simulink model "TEModel"  (Simulink 8.6)
settings: Solver=ode1  SolverMode=SingleTasking  StartTime=0.0  StopTime=72  FixedStep=Ts_base  MaxStep=Ts_base  MinStep=1e-6  RelTol=1e-6
PreLoadFcn:
  | initModel
StopFcn:
  | TEplot
undefined symbols (not defined in the file): Ts_base, Ts_save
libraries: TElib x45
(part 7 of 9)

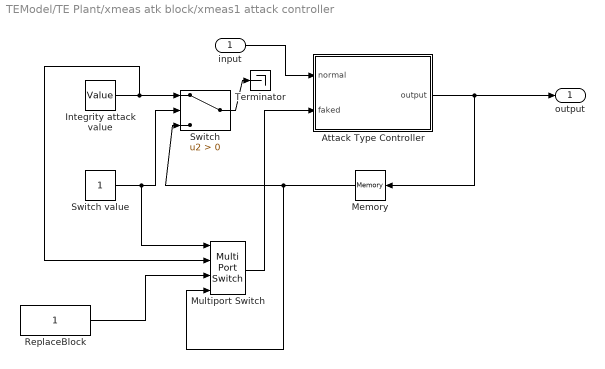
== system TEModel/TE Plant/xmeas atk block/xmeas1 attack controller ==
  input : Inport
  Attack Type Controller : Subsystem  Variant=on  OverrideUsingVariant=normal_forward_controller  mask{atkMode=No attack, start=1, duration=duration}
      mask prompts: atkMode "Attack Mode:"
      mask TypeOptions atkMode: No attack | Step attack | Interval attack | Periodical attack
      mask Callback atkMode:
      | switch get_param(gcb,'atkMode');
      |     case 'Step attack'
      |         set_param(gcb, 'OverrideUsingVariant', 'step_forward_controller');
      |     case 'Interval attack'
      |         set_param(gcb, 'OverrideUsingVariant', 'interval_forward_controller');
      |     case 'Periodical attack'
      |         set_param(gcb, 'OverrideUsingVariant', 'periodical_forward_controller');
      |     otherwise
      |         set_param(gcb, 'OverrideUsingVariant', 'normal_forward_controller');
      | end
      mask Display: eval(get_param([gcb '/' strrep(get_param(gcb, 'ActiveVariant'), '_', ' ')], 'MaskDisplay'));
  Integrity attack value : Constant  Value=Value
  Memory : Memory
  Multiport Switch : MultiPortSwitch
  ReplaceBlock : Constant
  Switch : Switch  Criteria=u2 > Threshold
  Switch value : Constant
  Terminator : Terminator
  output : Outport
  wires:
  Integrity attack value/1 -> Multiport Switch/2, Switch/1
  Attack Type Controller/1(output) -> Memory/1, output/1
  Switch value/1 -> Multiport Switch/1, Switch/2
  input/1 -> Attack Type Controller/1(normal)
  Memory/1 -> Multiport Switch/4, Switch/3
  Multiport Switch/1 -> Attack Type Controller/2(faked)
  Switch/1 -> Terminator/1
  ReplaceBlock/1 -> Multiport Switch/3

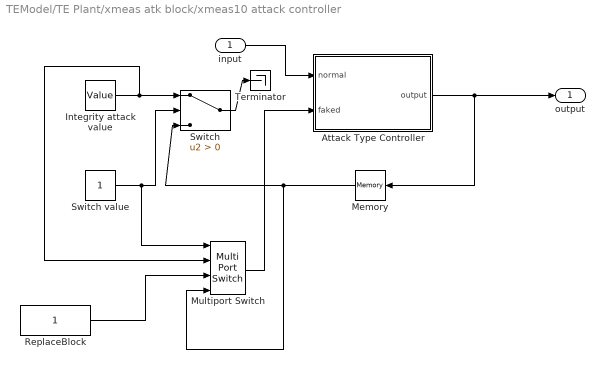
== system TEModel/TE Plant/xmeas atk block/xmeas10 attack controller ==
  input : Inport
  Attack Type Controller : Subsystem  Variant=on  OverrideUsingVariant=normal_forward_controller  mask{atkMode=No attack, start=1, duration=duration}
      mask prompts: atkMode "Attack Mode:"
      mask TypeOptions atkMode: No attack | Step attack | Interval attack | Periodical attack
      mask Callback atkMode:
      | switch get_param(gcb,'atkMode');
      |     case 'Step attack'
      |         set_param(gcb, 'OverrideUsingVariant', 'step_forward_controller');
      |     case 'Interval attack'
      |         set_param(gcb, 'OverrideUsingVariant', 'interval_forward_controller');
      |     case 'Periodical attack'
      |         set_param(gcb, 'OverrideUsingVariant', 'periodical_forward_controller');
      |     otherwise
      |         set_param(gcb, 'OverrideUsingVariant', 'normal_forward_controller');
      | end
      mask Display: eval(get_param([gcb '/' strrep(get_param(gcb, 'ActiveVariant'), '_', ' ')], 'MaskDisplay'));
  Integrity attack value : Constant  Value=Value
  Memory : Memory
  Multiport Switch : MultiPortSwitch
  ReplaceBlock : Constant
  Switch : Switch  Criteria=u2 > Threshold
  Switch value : Constant
  Terminator : Terminator
  output : Outport
  wires:
  Integrity attack value/1 -> Multiport Switch/2, Switch/1
  Attack Type Controller/1(output) -> Memory/1, output/1
  Switch value/1 -> Multiport Switch/1, Switch/2
  input/1 -> Attack Type Controller/1(normal)
  Memory/1 -> Multiport Switch/4, Switch/3
  Multiport Switch/1 -> Attack Type Controller/2(faked)
  Switch/1 -> Terminator/1
  ReplaceBlock/1 -> Multiport Switch/3

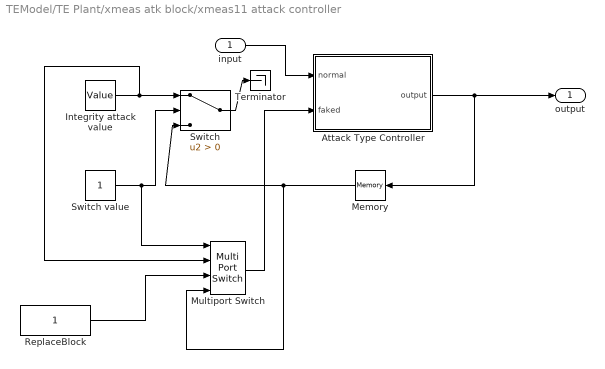
== system TEModel/TE Plant/xmeas atk block/xmeas11 attack controller ==
  input : Inport
  Attack Type Controller : Subsystem  Variant=on  OverrideUsingVariant=normal_forward_controller  mask{atkMode=No attack, start=1, duration=duration}
      mask prompts: atkMode "Attack Mode:"
      mask TypeOptions atkMode: No attack | Step attack | Interval attack | Periodical attack
      mask Callback atkMode:
      | switch get_param(gcb,'atkMode');
      |     case 'Step attack'
      |         set_param(gcb, 'OverrideUsingVariant', 'step_forward_controller');
      |     case 'Interval attack'
      |         set_param(gcb, 'OverrideUsingVariant', 'interval_forward_controller');
      |     case 'Periodical attack'
      |         set_param(gcb, 'OverrideUsingVariant', 'periodical_forward_controller');
      |     otherwise
      |         set_param(gcb, 'OverrideUsingVariant', 'normal_forward_controller');
      | end
      mask Display: eval(get_param([gcb '/' strrep(get_param(gcb, 'ActiveVariant'), '_', ' ')], 'MaskDisplay'));
  Integrity attack value : Constant  Value=Value
  Memory : Memory
  Multiport Switch : MultiPortSwitch
  ReplaceBlock : Constant
  Switch : Switch  Criteria=u2 > Threshold
  Switch value : Constant
  Terminator : Terminator
  output : Outport
  wires:
  Integrity attack value/1 -> Multiport Switch/2, Switch/1
  Attack Type Controller/1(output) -> Memory/1, output/1
  Switch value/1 -> Multiport Switch/1, Switch/2
  input/1 -> Attack Type Controller/1(normal)
  Memory/1 -> Multiport Switch/4, Switch/3
  Multiport Switch/1 -> Attack Type Controller/2(faked)
  Switch/1 -> Terminator/1
  ReplaceBlock/1 -> Multiport Switch/3

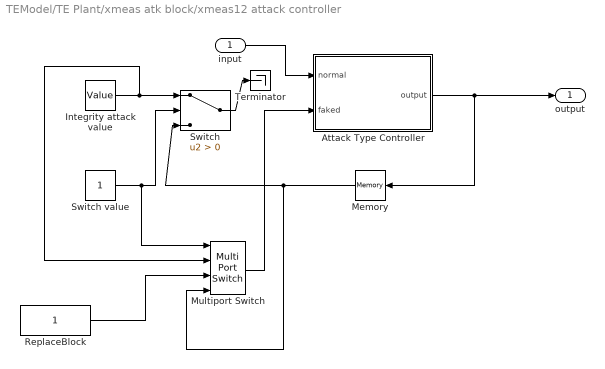
== system TEModel/TE Plant/xmeas atk block/xmeas12 attack controller ==
  input : Inport
  Attack Type Controller : Subsystem  Variant=on  OverrideUsingVariant=normal_forward_controller  mask{atkMode=No attack, start=1, duration=duration}
      mask prompts: atkMode "Attack Mode:"
      mask TypeOptions atkMode: No attack | Step attack | Interval attack | Periodical attack
      mask Callback atkMode:
      | switch get_param(gcb,'atkMode');
      |     case 'Step attack'
      |         set_param(gcb, 'OverrideUsingVariant', 'step_forward_controller');
      |     case 'Interval attack'
      |         set_param(gcb, 'OverrideUsingVariant', 'interval_forward_controller');
      |     case 'Periodical attack'
      |         set_param(gcb, 'OverrideUsingVariant', 'periodical_forward_controller');
      |     otherwise
      |         set_param(gcb, 'OverrideUsingVariant', 'normal_forward_controller');
      | end
      mask Display: eval(get_param([gcb '/' strrep(get_param(gcb, 'ActiveVariant'), '_', ' ')], 'MaskDisplay'));
  Integrity attack value : Constant  Value=Value
  Memory : Memory
  Multiport Switch : MultiPortSwitch
  ReplaceBlock : Constant
  Switch : Switch  Criteria=u2 > Threshold
  Switch value : Constant
  Terminator : Terminator
  output : Outport
  wires:
  Integrity attack value/1 -> Multiport Switch/2, Switch/1
  Attack Type Controller/1(output) -> Memory/1, output/1
  Switch value/1 -> Multiport Switch/1, Switch/2
  input/1 -> Attack Type Controller/1(normal)
  Memory/1 -> Multiport Switch/4, Switch/3
  Multiport Switch/1 -> Attack Type Controller/2(faked)
  Switch/1 -> Terminator/1
  ReplaceBlock/1 -> Multiport Switch/3

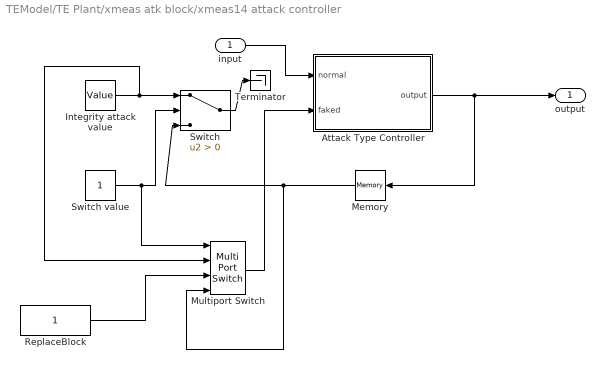
== system TEModel/TE Plant/xmeas atk block/xmeas14 attack controller ==
  input : Inport
  Attack Type Controller : Subsystem  Variant=on  OverrideUsingVariant=normal_forward_controller  mask{atkMode=No attack, start=1, duration=duration}
      mask prompts: atkMode "Attack Mode:"
      mask TypeOptions atkMode: No attack | Step attack | Interval attack | Periodical attack
      mask Callback atkMode:
      | switch get_param(gcb,'atkMode');
      |     case 'Step attack'
      |         set_param(gcb, 'OverrideUsingVariant', 'step_forward_controller');
      |     case 'Interval attack'
      |         set_param(gcb, 'OverrideUsingVariant', 'interval_forward_controller');
      |     case 'Periodical attack'
      |         set_param(gcb, 'OverrideUsingVariant', 'periodical_forward_controller');
      |     otherwise
      |         set_param(gcb, 'OverrideUsingVariant', 'normal_forward_controller');
      | end
      mask Display: eval(get_param([gcb '/' strrep(get_param(gcb, 'ActiveVariant'), '_', ' ')], 'MaskDisplay'));
  Integrity attack value : Constant  Value=Value
  Memory : Memory
  Multiport Switch : MultiPortSwitch
  ReplaceBlock : Constant
  Switch : Switch  Criteria=u2 > Threshold
  Switch value : Constant
  Terminator : Terminator
  output : Outport
  wires:
  Integrity attack value/1 -> Multiport Switch/2, Switch/1
  Attack Type Controller/1(output) -> Memory/1, output/1
  Switch value/1 -> Multiport Switch/1, Switch/2
  input/1 -> Attack Type Controller/1(normal)
  Memory/1 -> Multiport Switch/4, Switch/3
  Multiport Switch/1 -> Attack Type Controller/2(faked)
  Switch/1 -> Terminator/1
  ReplaceBlock/1 -> Multiport Switch/3

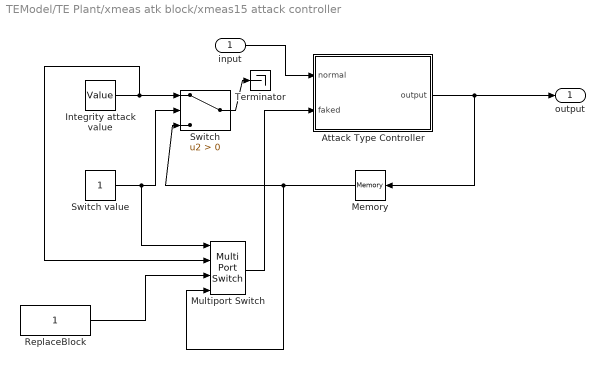
== system TEModel/TE Plant/xmeas atk block/xmeas15 attack controller ==
  input : Inport
  Attack Type Controller : Subsystem  Variant=on  OverrideUsingVariant=normal_forward_controller  mask{atkMode=No attack, start=1, duration=duration}
      mask prompts: atkMode "Attack Mode:"
      mask TypeOptions atkMode: No attack | Step attack | Interval attack | Periodical attack
      mask Callback atkMode:
      | switch get_param(gcb,'atkMode');
      |     case 'Step attack'
      |         set_param(gcb, 'OverrideUsingVariant', 'step_forward_controller');
      |     case 'Interval attack'
      |         set_param(gcb, 'OverrideUsingVariant', 'interval_forward_controller');
      |     case 'Periodical attack'
      |         set_param(gcb, 'OverrideUsingVariant', 'periodical_forward_controller');
      |     otherwise
      |         set_param(gcb, 'OverrideUsingVariant', 'normal_forward_controller');
      | end
      mask Display: eval(get_param([gcb '/' strrep(get_param(gcb, 'ActiveVariant'), '_', ' ')], 'MaskDisplay'));
  Integrity attack value : Constant  Value=Value
  Memory : Memory
  Multiport Switch : MultiPortSwitch
  ReplaceBlock : Constant
  Switch : Switch  Criteria=u2 > Threshold
  Switch value : Constant
  Terminator : Terminator
  output : Outport
  wires:
  Integrity attack value/1 -> Multiport Switch/2, Switch/1
  Attack Type Controller/1(output) -> Memory/1, output/1
  Switch value/1 -> Multiport Switch/1, Switch/2
  input/1 -> Attack Type Controller/1(normal)
  Memory/1 -> Multiport Switch/4, Switch/3
  Multiport Switch/1 -> Attack Type Controller/2(faked)
  Switch/1 -> Terminator/1
  ReplaceBlock/1 -> Multiport Switch/3

== system TEModel/TE Plant/xmeas atk block/xmeas17 attack controller ==
  input : Inport
  Attack Type Controller : Subsystem  Variant=on  OverrideUsingVariant=normal_forward_controller  mask{atkMode=No attack, start=1, duration=duration}
      mask prompts: atkMode "Attack Mode:"
      mask TypeOptions atkMode: No attack | Step attack | Interval attack | Periodical attack
      mask Callback atkMode:
      | switch get_param(gcb,'atkMode');
      |     case 'Step attack'
      |         set_param(gcb, 'OverrideUsingVariant', 'step_forward_controller');
      |     case 'Interval attack'
      |         set_param(gcb, 'OverrideUsingVariant', 'interval_forward_controller');
      |     case 'Periodical attack'
      |         set_param(gcb, 'OverrideUsingVariant', 'periodical_forward_controller');
      |     otherwise
      |         set_param(gcb, 'OverrideUsingVariant', 'normal_forward_controller');
      | end
      mask Display: eval(get_param([gcb '/' strrep(get_param(gcb, 'ActiveVariant'), '_', ' ')], 'MaskDisplay'));
  Integrity attack value : Constant  Value=Value
  Memory : Memory
  Multiport Switch : MultiPortSwitch
  ReplaceBlock : Constant
  Switch : Switch  Criteria=u2 > Threshold
  Switch value : Constant
  Terminator : Terminator
  output : Outport
  wires:
  Integrity attack value/1 -> Multiport Switch/2, Switch/1
  Attack Type Controller/1(output) -> Memory/1, output/1
  Switch value/1 -> Multiport Switch/1, Switch/2
  input/1 -> Attack Type Controller/1(normal)
  Memory/1 -> Multiport Switch/4, Switch/3
  Multiport Switch/1 -> Attack Type Controller/2(faked)
  Switch/1 -> Terminator/1
  ReplaceBlock/1 -> Multiport Switch/3

== system TEModel/TE Plant/xmeas atk block/xmeas2 attack controller ==
  input : Inport
  Attack Type Controller : Subsystem  Variant=on  OverrideUsingVariant=normal_forward_controller  mask{atkMode=No attack, start=1, duration=duration}
      mask prompts: atkMode "Attack Mode:"
      mask TypeOptions atkMode: No attack | Step attack | Interval attack | Periodical attack
      mask Callback atkMode:
      | switch get_param(gcb,'atkMode');
      |     case 'Step attack'
      |         set_param(gcb, 'OverrideUsingVariant', 'step_forward_controller');
      |     case 'Interval attack'
      |         set_param(gcb, 'OverrideUsingVariant', 'interval_forward_controller');
      |     case 'Periodical attack'
      |         set_param(gcb, 'OverrideUsingVariant', 'periodical_forward_controller');
      |     otherwise
      |         set_param(gcb, 'OverrideUsingVariant', 'normal_forward_controller');
      | end
      mask Display: eval(get_param([gcb '/' strrep(get_param(gcb, 'ActiveVariant'), '_', ' ')], 'MaskDisplay'));
  Integrity attack value : Constant  Value=Value
  Memory : Memory
  Multiport Switch : MultiPortSwitch
  ReplaceBlock : Constant
  Switch : Switch  Criteria=u2 > Threshold
  Switch value : Constant
  Terminator : Terminator
  output : Outport
  wires:
  Integrity attack value/1 -> Multiport Switch/2, Switch/1
  Attack Type Controller/1(output) -> Memory/1, output/1
  Switch value/1 -> Multiport Switch/1, Switch/2
  input/1 -> Attack Type Controller/1(normal)
  Memory/1 -> Multiport Switch/4, Switch/3
  Multiport Switch/1 -> Attack Type Controller/2(faked)
  Switch/1 -> Terminator/1
  ReplaceBlock/1 -> Multiport Switch/3

== system TEModel/TE Plant/xmeas atk block/xmeas3 attack controller ==
  input : Inport
  Attack Type Controller : Subsystem  Variant=on  OverrideUsingVariant=normal_forward_controller  mask{atkMode=No attack, start=1, duration=duration}
      mask prompts: atkMode "Attack Mode:"
      mask TypeOptions atkMode: No attack | Step attack | Interval attack | Periodical attack
      mask Callback atkMode:
      | switch get_param(gcb,'atkMode');
      |     case 'Step attack'
      |         set_param(gcb, 'OverrideUsingVariant', 'step_forward_controller');
      |     case 'Interval attack'
      |         set_param(gcb, 'OverrideUsingVariant', 'interval_forward_controller');
      |     case 'Periodical attack'
      |         set_param(gcb, 'OverrideUsingVariant', 'periodical_forward_controller');
      |     otherwise
      |         set_param(gcb, 'OverrideUsingVariant', 'normal_forward_controller');
      | end
      mask Display: eval(get_param([gcb '/' strrep(get_param(gcb, 'ActiveVariant'), '_', ' ')], 'MaskDisplay'));
  Integrity attack value : Constant  Value=Value
  Memory : Memory
  Multiport Switch : MultiPortSwitch
  ReplaceBlock : Constant
  Switch : Switch  Criteria=u2 > Threshold
  Switch value : Constant
  Terminator : Terminator
  output : Outport
  wires:
  Integrity attack value/1 -> Multiport Switch/2, Switch/1
  Attack Type Controller/1(output) -> Memory/1, output/1
  Switch value/1 -> Multiport Switch/1, Switch/2
  input/1 -> Attack Type Controller/1(normal)
  Memory/1 -> Multiport Switch/4, Switch/3
  Multiport Switch/1 -> Attack Type Controller/2(faked)
  Switch/1 -> Terminator/1
  ReplaceBlock/1 -> Multiport Switch/3

== system TEModel/TE Plant/xmeas atk block/xmeas31 attack controller ==
  input : Inport
  Attack Type Controller : Subsystem  Variant=on  OverrideUsingVariant=normal_forward_controller  mask{atkMode=No attack, start=1, duration=duration}
      mask prompts: atkMode "Attack Mode:"
      mask TypeOptions atkMode: No attack | Step attack | Interval attack | Periodical attack
      mask Callback atkMode:
      | switch get_param(gcb,'atkMode');
      |     case 'Step attack'
      |         set_param(gcb, 'OverrideUsingVariant', 'step_forward_controller');
      |     case 'Interval attack'
      |         set_param(gcb, 'OverrideUsingVariant', 'interval_forward_controller');
      |     case 'Periodical attack'
      |         set_param(gcb, 'OverrideUsingVariant', 'periodical_forward_controller');
      |     otherwise
      |         set_param(gcb, 'OverrideUsingVariant', 'normal_forward_controller');
      | end
      mask Display: eval(get_param([gcb '/' strrep(get_param(gcb, 'ActiveVariant'), '_', ' ')], 'MaskDisplay'));
  Integrity attack value : Constant  Value=Value
  Memory : Memory
  Multiport Switch : MultiPortSwitch
  ReplaceBlock : Constant
  Switch : Switch  Criteria=u2 > Threshold
  Switch value : Constant
  Terminator : Terminator
  output : Outport
  wires:
  Integrity attack value/1 -> Multiport Switch/2, Switch/1
  Attack Type Controller/1(output) -> Memory/1, output/1
  Switch value/1 -> Multiport Switch/1, Switch/2
  input/1 -> Attack Type Controller/1(normal)
  Memory/1 -> Multiport Switch/4, Switch/3
  Multiport Switch/1 -> Attack Type Controller/2(faked)
  Switch/1 -> Terminator/1
  ReplaceBlock/1 -> Multiport Switch/3

== system TEModel/TE Plant/xmeas atk block/xmeas4 attack controller ==
  input : Inport
  Attack Type Controller : Subsystem  Variant=on  OverrideUsingVariant=normal_forward_controller  mask{atkMode=No attack, start=1, duration=duration}
      mask prompts: atkMode "Attack Mode:"
      mask TypeOptions atkMode: No attack | Step attack | Interval attack | Periodical attack
      mask Callback atkMode:
      | switch get_param(gcb,'atkMode');
      |     case 'Step attack'
      |         set_param(gcb, 'OverrideUsingVariant', 'step_forward_controller');
      |     case 'Interval attack'
      |         set_param(gcb, 'OverrideUsingVariant', 'interval_forward_controller');
      |     case 'Periodical attack'
      |         set_param(gcb, 'OverrideUsingVariant', 'periodical_forward_controller');
      |     otherwise
      |         set_param(gcb, 'OverrideUsingVariant', 'normal_forward_controller');
      | end
      mask Display: eval(get_param([gcb '/' strrep(get_param(gcb, 'ActiveVariant'), '_', ' ')], 'MaskDisplay'));
  Integrity attack value : Constant  Value=Value
  Memory : Memory
  Multiport Switch : MultiPortSwitch
  ReplaceBlock : Constant
  Switch : Switch  Criteria=u2 > Threshold
  Switch value : Constant
  Terminator : Terminator
  output : Outport
  wires:
  Integrity attack value/1 -> Multiport Switch/2, Switch/1
  Attack Type Controller/1(output) -> Memory/1, output/1
  Switch value/1 -> Multiport Switch/1, Switch/2
  input/1 -> Attack Type Controller/1(normal)
  Memory/1 -> Multiport Switch/4, Switch/3
  Multiport Switch/1 -> Attack Type Controller/2(faked)
  Switch/1 -> Terminator/1
  ReplaceBlock/1 -> Multiport Switch/3

== system TEModel/TE Plant/xmeas atk block/xmeas40 attack controller ==
  input : Inport
  Attack Type Controller : Subsystem  Variant=on  OverrideUsingVariant=normal_forward_controller  mask{atkMode=No attack, start=1, duration=duration}
      mask prompts: atkMode "Attack Mode:"
      mask TypeOptions atkMode: No attack | Step attack | Interval attack | Periodical attack
      mask Callback atkMode:
      | switch get_param(gcb,'atkMode');
      |     case 'Step attack'
      |         set_param(gcb, 'OverrideUsingVariant', 'step_forward_controller');
      |     case 'Interval attack'
      |         set_param(gcb, 'OverrideUsingVariant', 'interval_forward_controller');
      |     case 'Periodical attack'
      |         set_param(gcb, 'OverrideUsingVariant', 'periodical_forward_controller');
      |     otherwise
      |         set_param(gcb, 'OverrideUsingVariant', 'normal_forward_controller');
      | end
      mask Display: eval(get_param([gcb '/' strrep(get_param(gcb, 'ActiveVariant'), '_', ' ')], 'MaskDisplay'));
  Integrity attack value : Constant  Value=Value
  Memory : Memory
  Multiport Switch : MultiPortSwitch
  ReplaceBlock : Constant
  Switch : Switch  Criteria=u2 > Threshold
  Switch value : Constant
  Terminator : Terminator
  output : Outport
  wires:
  Integrity attack value/1 -> Multiport Switch/2, Switch/1
  Attack Type Controller/1(output) -> Memory/1, output/1
  Switch value/1 -> Multiport Switch/1, Switch/2
  input/1 -> Attack Type Controller/1(normal)
  Memory/1 -> Multiport Switch/4, Switch/3
  Multiport Switch/1 -> Attack Type Controller/2(faked)
  Switch/1 -> Terminator/1
  ReplaceBlock/1 -> Multiport Switch/3

== system TEModel/TE Plant/xmeas atk block/xmeas5 attack controller ==
  input : Inport
  Attack Type Controller : Subsystem  Variant=on  OverrideUsingVariant=normal_forward_controller  mask{atkMode=No attack, start=1, duration=duration}
      mask prompts: atkMode "Attack Mode:"
      mask TypeOptions atkMode: No attack | Step attack | Interval attack | Periodical attack
      mask Callback atkMode:
      | switch get_param(gcb,'atkMode');
      |     case 'Step attack'
      |         set_param(gcb, 'OverrideUsingVariant', 'step_forward_controller');
      |     case 'Interval attack'
      |         set_param(gcb, 'OverrideUsingVariant', 'interval_forward_controller');
      |     case 'Periodical attack'
      |         set_param(gcb, 'OverrideUsingVariant', 'periodical_forward_controller');
      |     otherwise
      |         set_param(gcb, 'OverrideUsingVariant', 'normal_forward_controller');
      | end
      mask Display: eval(get_param([gcb '/' strrep(get_param(gcb, 'ActiveVariant'), '_', ' ')], 'MaskDisplay'));
  Integrity attack value : Constant  Value=Value
  Memory : Memory
  Multiport Switch : MultiPortSwitch
  ReplaceBlock : Constant
  Switch : Switch  Criteria=u2 > Threshold
  Switch value : Constant
  Terminator : Terminator
  output : Outport
  wires:
  Integrity attack value/1 -> Multiport Switch/2, Switch/1
  Attack Type Controller/1(output) -> Memory/1, output/1
  Switch value/1 -> Multiport Switch/1, Switch/2
  input/1 -> Attack Type Controller/1(normal)
  Memory/1 -> Multiport Switch/4, Switch/3
  Multiport Switch/1 -> Attack Type Controller/2(faked)
  Switch/1 -> Terminator/1
  ReplaceBlock/1 -> Multiport Switch/3

== system TEModel/TE Plant/xmeas atk block/xmeas7 attack controller ==
  input : Inport
  Attack Type Controller : Subsystem  Variant=on  OverrideUsingVariant=normal_forward_controller  mask{atkMode=No attack, start=1, duration=duration}
      mask prompts: atkMode "Attack Mode:"
      mask TypeOptions atkMode: No attack | Step attack | Interval attack | Periodical attack
      mask Callback atkMode:
      | switch get_param(gcb,'atkMode');
      |     case 'Step attack'
      |         set_param(gcb, 'OverrideUsingVariant', 'step_forward_controller');
      |     case 'Interval attack'
      |         set_param(gcb, 'OverrideUsingVariant', 'interval_forward_controller');
      |     case 'Periodical attack'
      |         set_param(gcb, 'OverrideUsingVariant', 'periodical_forward_controller');
      |     otherwise
      |         set_param(gcb, 'OverrideUsingVariant', 'normal_forward_controller');
      | end
      mask Display: eval(get_param([gcb '/' strrep(get_param(gcb, 'ActiveVariant'), '_', ' ')], 'MaskDisplay'));
  Integrity attack value : Constant  Value=Value
  Memory : Memory
  Multiport Switch : MultiPortSwitch
  ReplaceBlock : Constant
  Switch : Switch  Criteria=u2 > Threshold
  Switch value : Constant
  Terminator : Terminator
  output : Outport
  wires:
  Integrity attack value/1 -> Multiport Switch/2, Switch/1
  Attack Type Controller/1(output) -> Memory/1, output/1
  Switch value/1 -> Multiport Switch/1, Switch/2
  input/1 -> Attack Type Controller/1(normal)
  Memory/1 -> Multiport Switch/4, Switch/3
  Multiport Switch/1 -> Attack Type Controller/2(faked)
  Switch/1 -> Terminator/1
  ReplaceBlock/1 -> Multiport Switch/3

== system TEModel/TE Plant/xmeas atk block/xmeas8 attack controller ==
  input : Inport
  Attack Type Controller : Subsystem  Variant=on  OverrideUsingVariant=normal_forward_controller  mask{atkMode=No attack, start=1, duration=duration}
      mask prompts: atkMode "Attack Mode:"
      mask TypeOptions atkMode: No attack | Step attack | Interval attack | Periodical attack
      mask Callback atkMode:
      | switch get_param(gcb,'atkMode');
      |     case 'Step attack'
      |         set_param(gcb, 'OverrideUsingVariant', 'step_forward_controller');
      |     case 'Interval attack'
      |         set_param(gcb, 'OverrideUsingVariant', 'interval_forward_controller');
      |     case 'Periodical attack'
      |         set_param(gcb, 'OverrideUsingVariant', 'periodical_forward_controller');
      |     otherwise
      |         set_param(gcb, 'OverrideUsingVariant', 'normal_forward_controller');
      | end
      mask Display: eval(get_param([gcb '/' strrep(get_param(gcb, 'ActiveVariant'), '_', ' ')], 'MaskDisplay'));
  Integrity attack value : Constant  Value=Value
  Memory : Memory
  Multiport Switch : MultiPortSwitch
  ReplaceBlock : Constant
  Switch : Switch  Criteria=u2 > Threshold
  Switch value : Constant
  Terminator : Terminator
  output : Outport
  wires:
  Integrity attack value/1 -> Multiport Switch/2, Switch/1
  Attack Type Controller/1(output) -> Memory/1, output/1
  Switch value/1 -> Multiport Switch/1, Switch/2
  input/1 -> Attack Type Controller/1(normal)
  Memory/1 -> Multiport Switch/4, Switch/3
  Multiport Switch/1 -> Attack Type Controller/2(faked)
  Switch/1 -> Terminator/1
  ReplaceBlock/1 -> Multiport Switch/3

== system TEModel/TE Plant/xmeas atk block/xmeas9 attack controller ==
  input : Inport
  Attack Type Controller : Subsystem  Variant=on  OverrideUsingVariant=normal_forward_controller  mask{atkMode=No attack, start=1, duration=duration}
      mask prompts: atkMode "Attack Mode:"
      mask TypeOptions atkMode: No attack | Step attack | Interval attack | Periodical attack
      mask Callback atkMode:
      | switch get_param(gcb,'atkMode');
      |     case 'Step attack'
      |         set_param(gcb, 'OverrideUsingVariant', 'step_forward_controller');
      |     case 'Interval attack'
      |         set_param(gcb, 'OverrideUsingVariant', 'interval_forward_controller');
      |     case 'Periodical attack'
      |         set_param(gcb, 'OverrideUsingVariant', 'periodical_forward_controller');
      |     otherwise
      |         set_param(gcb, 'OverrideUsingVariant', 'normal_forward_controller');
      | end
      mask Display: eval(get_param([gcb '/' strrep(get_param(gcb, 'ActiveVariant'), '_', ' ')], 'MaskDisplay'));
  Integrity attack value : Constant  Value=Value
  Memory : Memory
  Multiport Switch : MultiPortSwitch
  ReplaceBlock : Constant
  Switch : Switch  Criteria=u2 > Threshold
  Switch value : Constant
  Terminator : Terminator
  output : Outport
  wires:
  Integrity attack value/1 -> Multiport Switch/2, Switch/1
  Attack Type Controller/1(output) -> Memory/1, output/1
  Switch value/1 -> Multiport Switch/1, Switch/2
  input/1 -> Attack Type Controller/1(normal)
  Memory/1 -> Multiport Switch/4, Switch/3
  Multiport Switch/1 -> Attack Type Controller/2(faked)
  Switch/1 -> Terminator/1
  ReplaceBlock/1 -> Multiport Switch/3

== system TEModel/TE Plant/xmv atk block/xmv1 attack controller ==
  input : Inport
  Attack Type Controller : Subsystem  Variant=on  OverrideUsingVariant=normal_forward_controller  mask{atkMode=No attack, start=1, duration=duration}
      mask prompts: atkMode "Attack Mode:"
      mask TypeOptions atkMode: No attack | Step attack | Interval attack | Periodical attack
      mask Callback atkMode:
      | switch get_param(gcb,'atkMode');
      |     case 'Step attack'
      |         set_param(gcb, 'OverrideUsingVariant', 'step_forward_controller');
      |     case 'Interval attack'
      |         set_param(gcb, 'OverrideUsingVariant', 'interval_forward_controller');
      |     case 'Periodical attack'
      |         set_param(gcb, 'OverrideUsingVariant', 'periodical_forward_controller');
      |     otherwise
      |         set_param(gcb, 'OverrideUsingVariant', 'normal_forward_controller');
      | end
      mask Display: eval(get_param([gcb '/' strrep(get_param(gcb, 'ActiveVariant'), '_', ' ')], 'MaskDisplay'));
  Integrity attack value : Constant  Value=Value
  Memory : Memory
  Multiport Switch : MultiPortSwitch
  ReplaceBlock : Constant
  Switch : Switch  Criteria=u2 > Threshold
  Switch value : Constant
  Terminator : Terminator
  output : Outport
  wires:
  Integrity attack value/1 -> Multiport Switch/2, Switch/1
  Attack Type Controller/1(output) -> Memory/1, output/1
  Switch value/1 -> Multiport Switch/1, Switch/2
  input/1 -> Attack Type Controller/1(normal)
  Memory/1 -> Multiport Switch/4, Switch/3
  Multiport Switch/1 -> Attack Type Controller/2(faked)
  Switch/1 -> Terminator/1
  ReplaceBlock/1 -> Multiport Switch/3

== system TEModel/TE Plant/xmv atk block/xmv10 attack controller ==
  input : Inport
  Attack Type Controller : Subsystem  Variant=on  OverrideUsingVariant=normal_forward_controller  mask{atkMode=No attack, start=1, duration=duration}
      mask prompts: atkMode "Attack Mode:"
      mask TypeOptions atkMode: No attack | Step attack | Interval attack | Periodical attack
      mask Callback atkMode:
      | switch get_param(gcb,'atkMode');
      |     case 'Step attack'
      |         set_param(gcb, 'OverrideUsingVariant', 'step_forward_controller');
      |     case 'Interval attack'
      |         set_param(gcb, 'OverrideUsingVariant', 'interval_forward_controller');
      |     case 'Periodical attack'
      |         set_param(gcb, 'OverrideUsingVariant', 'periodical_forward_controller');
      |     otherwise
      |         set_param(gcb, 'OverrideUsingVariant', 'normal_forward_controller');
      | end
      mask Display: eval(get_param([gcb '/' strrep(get_param(gcb, 'ActiveVariant'), '_', ' ')], 'MaskDisplay'));
  Integrity attack value : Constant  Value=Value
  Memory : Memory
  Multiport Switch : MultiPortSwitch
  ReplaceBlock : Constant
  Switch : Switch  Criteria=u2 > Threshold
  Switch value : Constant
  Terminator : Terminator
  output : Outport
  wires:
  Integrity attack value/1 -> Multiport Switch/2, Switch/1
  Attack Type Controller/1(output) -> Memory/1, output/1
  Switch value/1 -> Multiport Switch/1, Switch/2
  input/1 -> Attack Type Controller/1(normal)
  Memory/1 -> Multiport Switch/4, Switch/3
  Multiport Switch/1 -> Attack Type Controller/2(faked)
  Switch/1 -> Terminator/1
  ReplaceBlock/1 -> Multiport Switch/3

== system TEModel/TE Plant/xmv atk block/xmv11 attack controller ==
  input : Inport
  Attack Type Controller : Subsystem  Variant=on  OverrideUsingVariant=normal_forward_controller  mask{atkMode=No attack, start=1, duration=duration}
      mask prompts: atkMode "Attack Mode:"
      mask TypeOptions atkMode: No attack | Step attack | Interval attack | Periodical attack
      mask Callback atkMode:
      | switch get_param(gcb,'atkMode');
      |     case 'Step attack'
      |         set_param(gcb, 'OverrideUsingVariant', 'step_forward_controller');
      |     case 'Interval attack'
      |         set_param(gcb, 'OverrideUsingVariant', 'interval_forward_controller');
      |     case 'Periodical attack'
      |         set_param(gcb, 'OverrideUsingVariant', 'periodical_forward_controller');
      |     otherwise
      |         set_param(gcb, 'OverrideUsingVariant', 'normal_forward_controller');
      | end
      mask Display: eval(get_param([gcb '/' strrep(get_param(gcb, 'ActiveVariant'), '_', ' ')], 'MaskDisplay'));
  Integrity attack value : Constant  Value=Value
  Memory : Memory
  Multiport Switch : MultiPortSwitch
  ReplaceBlock : Constant
  Switch : Switch  Criteria=u2 > Threshold
  Switch value : Constant
  Terminator : Terminator
  output : Outport
  wires:
  Integrity attack value/1 -> Multiport Switch/2, Switch/1
  Attack Type Controller/1(output) -> Memory/1, output/1
  Switch value/1 -> Multiport Switch/1, Switch/2
  input/1 -> Attack Type Controller/1(normal)
  Memory/1 -> Multiport Switch/4, Switch/3
  Multiport Switch/1 -> Attack Type Controller/2(faked)
  Switch/1 -> Terminator/1
  ReplaceBlock/1 -> Multiport Switch/3

== system TEModel/TE Plant/xmv atk block/xmv12 attack controller ==
  input : Inport
  Attack Type Controller : Subsystem  Variant=on  OverrideUsingVariant=normal_forward_controller  mask{atkMode=No attack, start=1, duration=duration}
      mask prompts: atkMode "Attack Mode:"
      mask TypeOptions atkMode: No attack | Step attack | Interval attack | Periodical attack
      mask Callback atkMode:
      | switch get_param(gcb,'atkMode');
      |     case 'Step attack'
      |         set_param(gcb, 'OverrideUsingVariant', 'step_forward_controller');
      |     case 'Interval attack'
      |         set_param(gcb, 'OverrideUsingVariant', 'interval_forward_controller');
      |     case 'Periodical attack'
      |         set_param(gcb, 'OverrideUsingVariant', 'periodical_forward_controller');
      |     otherwise
      |         set_param(gcb, 'OverrideUsingVariant', 'normal_forward_controller');
      | end
      mask Display: eval(get_param([gcb '/' strrep(get_param(gcb, 'ActiveVariant'), '_', ' ')], 'MaskDisplay'));
  Integrity attack value : Constant  Value=Value
  Memory : Memory
  Multiport Switch : MultiPortSwitch
  ReplaceBlock : Constant
  Switch : Switch  Criteria=u2 > Threshold
  Switch value : Constant
  Terminator : Terminator
  output : Outport
  wires:
  Integrity attack value/1 -> Multiport Switch/2, Switch/1
  Attack Type Controller/1(output) -> Memory/1, output/1
  Switch value/1 -> Multiport Switch/1, Switch/2
  input/1 -> Attack Type Controller/1(normal)
  Memory/1 -> Multiport Switch/4, Switch/3
  Multiport Switch/1 -> Attack Type Controller/2(faked)
  Switch/1 -> Terminator/1
  ReplaceBlock/1 -> Multiport Switch/3

== system TEModel/TE Plant/xmv atk block/xmv2 attack controller ==
  input : Inport
  Attack Type Controller : Subsystem  Variant=on  OverrideUsingVariant=normal_forward_controller  mask{atkMode=No attack, start=1, duration=duration}
      mask prompts: atkMode "Attack Mode:"
      mask TypeOptions atkMode: No attack | Step attack | Interval attack | Periodical attack
      mask Callback atkMode:
      | switch get_param(gcb,'atkMode');
      |     case 'Step attack'
      |         set_param(gcb, 'OverrideUsingVariant', 'step_forward_controller');
      |     case 'Interval attack'
      |         set_param(gcb, 'OverrideUsingVariant', 'interval_forward_controller');
      |     case 'Periodical attack'
      |         set_param(gcb, 'OverrideUsingVariant', 'periodical_forward_controller');
      |     otherwise
      |         set_param(gcb, 'OverrideUsingVariant', 'normal_forward_controller');
      | end
      mask Display: eval(get_param([gcb '/' strrep(get_param(gcb, 'ActiveVariant'), '_', ' ')], 'MaskDisplay'));
  Integrity attack value : Constant  Value=Value
  Memory : Memory
  Multiport Switch : MultiPortSwitch
  ReplaceBlock : Constant
  Switch : Switch  Criteria=u2 > Threshold
  Switch value : Constant
  Terminator : Terminator
  output : Outport
  wires:
  Integrity attack value/1 -> Multiport Switch/2, Switch/1
  Attack Type Controller/1(output) -> Memory/1, output/1
  Switch value/1 -> Multiport Switch/1, Switch/2
  input/1 -> Attack Type Controller/1(normal)
  Memory/1 -> Multiport Switch/4, Switch/3
  Multiport Switch/1 -> Attack Type Controller/2(faked)
  Switch/1 -> Terminator/1
  ReplaceBlock/1 -> Multiport Switch/3

== system TEModel/TE Plant/xmv atk block/xmv3 attack controller ==
  input : Inport
  Attack Type Controller : Subsystem  Variant=on  OverrideUsingVariant=normal_forward_controller  mask{atkMode=No attack, start=14.2928, duration=duration}
      mask prompts: atkMode "Attack Mode:"
      mask TypeOptions atkMode: No attack | Step attack | Interval attack | Periodical attack
      mask Callback atkMode:
      | switch get_param(gcb,'atkMode');
      |     case 'Step attack'
      |         set_param(gcb, 'OverrideUsingVariant', 'step_forward_controller');
      |     case 'Interval attack'
      |         set_param(gcb, 'OverrideUsingVariant', 'interval_forward_controller');
      |     case 'Periodical attack'
      |         set_param(gcb, 'OverrideUsingVariant', 'periodical_forward_controller');
      |     otherwise
      |         set_param(gcb, 'OverrideUsingVariant', 'normal_forward_controller');
      | end
      mask Display: eval(get_param([gcb '/' strrep(get_param(gcb, 'ActiveVariant'), '_', ' ')], 'MaskDisplay'));
  Integrity attack value : Constant  Value=Value
  Memory : Memory
  Multiport Switch : MultiPortSwitch
  ReplaceBlock : Constant
  Switch : Switch  Criteria=u2 > Threshold
  Switch value : Constant  Value=3
  Terminator : Terminator
  output : Outport
  wires:
  Integrity attack value/1 -> Multiport Switch/2, Switch/1
  Attack Type Controller/1(output) -> Memory/1, output/1
  Switch value/1 -> Multiport Switch/1, Switch/2
  input/1 -> Attack Type Controller/1(normal)
  Memory/1 -> Multiport Switch/4, Switch/3
  Multiport Switch/1 -> Attack Type Controller/2(faked)
  Switch/1 -> Terminator/1
  ReplaceBlock/1 -> Multiport Switch/3

== system TEModel/TE Plant/xmv atk block/xmv4 attack controller ==
  input : Inport
  Attack Type Controller : Subsystem  Variant=on  OverrideUsingVariant=normal_forward_controller  mask{atkMode=No attack, start=1, duration=duration}
      mask prompts: atkMode "Attack Mode:"
      mask TypeOptions atkMode: No attack | Step attack | Interval attack | Periodical attack
      mask Callback atkMode:
      | switch get_param(gcb,'atkMode');
      |     case 'Step attack'
      |         set_param(gcb, 'OverrideUsingVariant', 'step_forward_controller');
      |     case 'Interval attack'
      |         set_param(gcb, 'OverrideUsingVariant', 'interval_forward_controller');
      |     case 'Periodical attack'
      |         set_param(gcb, 'OverrideUsingVariant', 'periodical_forward_controller');
      |     otherwise
      |         set_param(gcb, 'OverrideUsingVariant', 'normal_forward_controller');
      | end
      mask Display: eval(get_param([gcb '/' strrep(get_param(gcb, 'ActiveVariant'), '_', ' ')], 'MaskDisplay'));
  Integrity attack value : Constant  Value=Value
  Memory : Memory
  Multiport Switch : MultiPortSwitch
  ReplaceBlock : Constant
  Switch : Switch  Criteria=u2 > Threshold
  Switch value : Constant
  Terminator : Terminator
  output : Outport
  wires:
  Integrity attack value/1 -> Multiport Switch/2, Switch/1
  Attack Type Controller/1(output) -> Memory/1, output/1
  Switch value/1 -> Multiport Switch/1, Switch/2
  input/1 -> Attack Type Controller/1(normal)
  Memory/1 -> Multiport Switch/4, Switch/3
  Multiport Switch/1 -> Attack Type Controller/2(faked)
  Switch/1 -> Terminator/1
  ReplaceBlock/1 -> Multiport Switch/3

== system TEModel/TE Plant/xmv atk block/xmv5 attack controller ==
  input : Inport
  Attack Type Controller : Subsystem  Variant=on  OverrideUsingVariant=normal_forward_controller  mask{atkMode=No attack, start=1, duration=duration}
      mask prompts: atkMode "Attack Mode:"
      mask TypeOptions atkMode: No attack | Step attack | Interval attack | Periodical attack
      mask Callback atkMode:
      | switch get_param(gcb,'atkMode');
      |     case 'Step attack'
      |         set_param(gcb, 'OverrideUsingVariant', 'step_forward_controller');
      |     case 'Interval attack'
      |         set_param(gcb, 'OverrideUsingVariant', 'interval_forward_controller');
      |     case 'Periodical attack'
      |         set_param(gcb, 'OverrideUsingVariant', 'periodical_forward_controller');
      |     otherwise
      |         set_param(gcb, 'OverrideUsingVariant', 'normal_forward_controller');
      | end
      mask Display: eval(get_param([gcb '/' strrep(get_param(gcb, 'ActiveVariant'), '_', ' ')], 'MaskDisplay'));
  Integrity attack value : Constant  Value=Value
  Memory : Memory
  Multiport Switch : MultiPortSwitch
  ReplaceBlock : Constant
  Switch : Switch  Criteria=u2 > Threshold
  Switch value : Constant
  Terminator : Terminator
  output : Outport
  wires:
  Integrity attack value/1 -> Multiport Switch/2, Switch/1
  Attack Type Controller/1(output) -> Memory/1, output/1
  Switch value/1 -> Multiport Switch/1, Switch/2
  input/1 -> Attack Type Controller/1(normal)
  Memory/1 -> Multiport Switch/4, Switch/3
  Multiport Switch/1 -> Attack Type Controller/2(faked)
  Switch/1 -> Terminator/1
  ReplaceBlock/1 -> Multiport Switch/3

== system TEModel/TE Plant/xmv atk block/xmv6 attack controller ==
  input : Inport
  Attack Type Controller : Subsystem  Variant=on  OverrideUsingVariant=normal_forward_controller  mask{atkMode=No attack, start=1, duration=duration}
      mask prompts: atkMode "Attack Mode:"
      mask TypeOptions atkMode: No attack | Step attack | Interval attack | Periodical attack
      mask Callback atkMode:
      | switch get_param(gcb,'atkMode');
      |     case 'Step attack'
      |         set_param(gcb, 'OverrideUsingVariant', 'step_forward_controller');
      |     case 'Interval attack'
      |         set_param(gcb, 'OverrideUsingVariant', 'interval_forward_controller');
      |     case 'Periodical attack'
      |         set_param(gcb, 'OverrideUsingVariant', 'periodical_forward_controller');
      |     otherwise
      |         set_param(gcb, 'OverrideUsingVariant', 'normal_forward_controller');
      | end
      mask Display: eval(get_param([gcb '/' strrep(get_param(gcb, 'ActiveVariant'), '_', ' ')], 'MaskDisplay'));
  Integrity attack value : Constant  Value=Value
  Memory : Memory
  Multiport Switch : MultiPortSwitch
  ReplaceBlock : Constant
  Switch : Switch  Criteria=u2 > Threshold
  Switch value : Constant
  Terminator : Terminator
  output : Outport
  wires:
  Integrity attack value/1 -> Multiport Switch/2, Switch/1
  Attack Type Controller/1(output) -> Memory/1, output/1
  Switch value/1 -> Multiport Switch/1, Switch/2
  input/1 -> Attack Type Controller/1(normal)
  Memory/1 -> Multiport Switch/4, Switch/3
  Multiport Switch/1 -> Attack Type Controller/2(faked)
  Switch/1 -> Terminator/1
  ReplaceBlock/1 -> Multiport Switch/3

== system TEModel/TE Plant/xmv atk block/xmv7 attack controller ==
  input : Inport
  Attack Type Controller : Subsystem  Variant=on  OverrideUsingVariant=normal_forward_controller  mask{atkMode=No attack, start=1, duration=duration}
      mask prompts: atkMode "Attack Mode:"
      mask TypeOptions atkMode: No attack | Step attack | Interval attack | Periodical attack
      mask Callback atkMode:
      | switch get_param(gcb,'atkMode');
      |     case 'Step attack'
      |         set_param(gcb, 'OverrideUsingVariant', 'step_forward_controller');
      |     case 'Interval attack'
      |         set_param(gcb, 'OverrideUsingVariant', 'interval_forward_controller');
      |     case 'Periodical attack'
      |         set_param(gcb, 'OverrideUsingVariant', 'periodical_forward_controller');
      |     otherwise
      |         set_param(gcb, 'OverrideUsingVariant', 'normal_forward_controller');
      | end
      mask Display: eval(get_param([gcb '/' strrep(get_param(gcb, 'ActiveVariant'), '_', ' ')], 'MaskDisplay'));
  Integrity attack value : Constant  Value=Value
  Memory : Memory
  Multiport Switch : MultiPortSwitch
  ReplaceBlock : Constant
  Switch : Switch  Criteria=u2 > Threshold
  Switch value : Constant
  Terminator : Terminator
  output : Outport
  wires:
  Integrity attack value/1 -> Multiport Switch/2, Switch/1
  Attack Type Controller/1(output) -> Memory/1, output/1
  Switch value/1 -> Multiport Switch/1, Switch/2
  input/1 -> Attack Type Controller/1(normal)
  Memory/1 -> Multiport Switch/4, Switch/3
  Multiport Switch/1 -> Attack Type Controller/2(faked)
  Switch/1 -> Terminator/1
  ReplaceBlock/1 -> Multiport Switch/3

== system TEModel/TE Plant/xmv atk block/xmv8 attack controller ==
  input : Inport
  Attack Type Controller : Subsystem  Variant=on  OverrideUsingVariant=normal_forward_controller  mask{atkMode=No attack, start=1, duration=duration}
      mask prompts: atkMode "Attack Mode:"
      mask TypeOptions atkMode: No attack | Step attack | Interval attack | Periodical attack
      mask Callback atkMode:
      | switch get_param(gcb,'atkMode');
      |     case 'Step attack'
      |         set_param(gcb, 'OverrideUsingVariant', 'step_forward_controller');
      |     case 'Interval attack'
      |         set_param(gcb, 'OverrideUsingVariant', 'interval_forward_controller');
      |     case 'Periodical attack'
      |         set_param(gcb, 'OverrideUsingVariant', 'periodical_forward_controller');
      |     otherwise
      |         set_param(gcb, 'OverrideUsingVariant', 'normal_forward_controller');
      | end
      mask Display: eval(get_param([gcb '/' strrep(get_param(gcb, 'ActiveVariant'), '_', ' ')], 'MaskDisplay'));
  Integrity attack value : Constant  Value=Value
  Memory : Memory
  Multiport Switch : MultiPortSwitch
  ReplaceBlock : Constant
  Switch : Switch  Criteria=u2 > Threshold
  Switch value : Constant
  Terminator : Terminator
  output : Outport
  wires:
  Integrity attack value/1 -> Multiport Switch/2, Switch/1
  Attack Type Controller/1(output) -> Memory/1, output/1
  Switch value/1 -> Multiport Switch/1, Switch/2
  input/1 -> Attack Type Controller/1(normal)
  Memory/1 -> Multiport Switch/4, Switch/3
  Multiport Switch/1 -> Attack Type Controller/2(faked)
  Switch/1 -> Terminator/1
  ReplaceBlock/1 -> Multiport Switch/3

== system TEModel/TE Plant/xmv atk block/xmv9 attack controller ==
  input : Inport
  Attack Type Controller : Subsystem  Variant=on  OverrideUsingVariant=normal_forward_controller  mask{atkMode=No attack, start=1, duration=duration}
      mask prompts: atkMode "Attack Mode:"
      mask TypeOptions atkMode: No attack | Step attack | Interval attack | Periodical attack
      mask Callback atkMode:
      | switch get_param(gcb,'atkMode');
      |     case 'Step attack'
      |         set_param(gcb, 'OverrideUsingVariant', 'step_forward_controller');
      |     case 'Interval attack'
      |         set_param(gcb, 'OverrideUsingVariant', 'interval_forward_controller');
      |     case 'Periodical attack'
      |         set_param(gcb, 'OverrideUsingVariant', 'periodical_forward_controller');
      |     otherwise
      |         set_param(gcb, 'OverrideUsingVariant', 'normal_forward_controller');
      | end
      mask Display: eval(get_param([gcb '/' strrep(get_param(gcb, 'ActiveVariant'), '_', ' ')], 'MaskDisplay'));
  Integrity attack value : Constant  Value=Value
  Memory : Memory
  Multiport Switch : MultiPortSwitch
  ReplaceBlock : Constant
  Switch : Switch  Criteria=u2 > Threshold
  Switch value : Constant
  Terminator : Terminator
  output : Outport
  wires:
  Integrity attack value/1 -> Multiport Switch/2, Switch/1
  Attack Type Controller/1(output) -> Memory/1, output/1
  Switch value/1 -> Multiport Switch/1, Switch/2
  input/1 -> Attack Type Controller/1(normal)
  Memory/1 -> Multiport Switch/4, Switch/3
  Multiport Switch/1 -> Attack Type Controller/2(faked)
  Switch/1 -> Terminator/1
  ReplaceBlock/1 -> Multiport Switch/3

== system TEModel/TE Plant/xmeas atk block/xmeas1 attack controller/Attack Type Controller ==
  note: 1) Only subsystems can be added as variant choices at this level
      | 2) Blocks cannot be connected at this level as connectivity is
      | automatically determined at simulation, based on the active variant
  normal : Inport
  faked : Inport  Port=2
  interval forward controller : Subsystem  VariantControl=interval_forward_controller
      mask Display:
      | disp('IFC')
      | port_label('input', 1, 'normal in')
      | port_label('input', 2, 'faked in')
      | port_label('output', 1, 'out')
  normal forward controller : Subsystem  VariantControl=normal_forward_controller
      mask Display:
      | disp('NFC')
      | port_label('input', 1, 'normal in')
      | port_label('input', 2, 'faked in')
      | port_label('output', 1, 'out')
  periodical forward controller : Subsystem  VariantControl=periodical_forward_controller
      mask Display:
      | disp('PFC')
      | port_label('input', 1, 'normal in')
      | port_label('input', 2, 'faked in')
      | port_label('output', 1, 'out')
  step forward controller : Subsystem  VariantControl=step_forward_controller
      mask Display:
      | disp('SFC')
      | port_label('input', 1, 'normal in')
      | port_label('input', 2, 'faked in')
      | port_label('output', 1, 'out')
  output : Outport

== system TEModel/TE Plant/xmeas atk block/xmeas10 attack controller/Attack Type Controller ==
  note: 1) Only subsystems can be added as variant choices at this level
      | 2) Blocks cannot be connected at this level as connectivity is
      | automatically determined at simulation, based on the active variant
  normal : Inport
  faked : Inport  Port=2
  interval forward controller : Subsystem  VariantControl=interval_forward_controller
      mask Display:
      | disp('IFC')
      | port_label('input', 1, 'normal in')
      | port_label('input', 2, 'faked in')
      | port_label('output', 1, 'out')
  normal forward controller : Subsystem  VariantControl=normal_forward_controller
      mask Display:
      | disp('NFC')
      | port_label('input', 1, 'normal in')
      | port_label('input', 2, 'faked in')
      | port_label('output', 1, 'out')
  periodical forward controller : Subsystem  VariantControl=periodical_forward_controller
      mask Display:
      | disp('PFC')
      | port_label('input', 1, 'normal in')
      | port_label('input', 2, 'faked in')
      | port_label('output', 1, 'out')
  step forward controller : Subsystem  VariantControl=step_forward_controller
      mask Display:
      | disp('SFC')
      | port_label('input', 1, 'normal in')
      | port_label('input', 2, 'faked in')
      | port_label('output', 1, 'out')
  output : Outport
